simulink model "STATCOM_Model"  (R2017a)
settings: Solver=FixedStepDiscrete  StartTime=0.0  StopTime=3  RelTol=1e-4  EnableMultiTasking=on
PreLoadFcn:
  | power_converters_init;
values from neighbouring files (symbols this model uses):
  Clink_3L = Pnom_dc_3L*H_3L*2 /Vnom_dc_3L^2    (= 2.77008310249e-05)    [STATCOM_init.m]
  Fnom = 50    [STATCOM_init.m]
  LimitL_Ireg_3L = -1.5    [STATCOM_init.m]
  LimitU_Ireg_3L = 1.5    [STATCOM_init.m]
  Lxfo_3L = 0.10    (= 0.1)    [STATCOM_init.m]
  Pnom_3L = Pnom_dc_3L    (= 50000000)    [STATCOM_init.m]
  Pnom_dc_3L = 50e6    (= 50000000)    [STATCOM_init.m]
  Rxfo_3L = 0.10/30    (= 0.00333333333333)    [STATCOM_init.m]
  Ts_Control = 50e-6    (= 5e-05)    [STATCOM_init.m]
  Ts_Power = Ts_PWM    (= 5e-06)    [STATCOM_init.m]
  Ts_PWM = 5e-6    (= 5e-06)    [STATCOM_init.m]
  Vnom_dc_3L = 380e3    (= 380000)    [STATCOM_init.m]
  Vnom_grid = 230e3    (= 230000)    [STATCOM_init.m]
  Vnom_prim_3L = Vnom_grid    (= 230000)    [STATCOM_init.m]
  Vnom_sec_3L = 0.5*Vnom_dc_3L/sqrt(2)*sqrt(3)*m_nom_3L    [STATCOM_init.m]
undefined symbols (not defined in the file or in its folder): D1, Delta, DiscIntNeverNeededParam
undefined symbols (not defined in the file): Ki_Ireg_3L, Ki_VDCreg_3L, Kp_Ireg_3L, Kp_VDCreg_3L, LimitL_VDCreg_3L, LimitU_VDCreg_3L
libraries: powerlib x23, powerlib_meascontrol x11, powerlib_extras x1
(part 2 of 2)

== system STATCOM_Model/Control System  ==
  Statcom Control : Subsystem

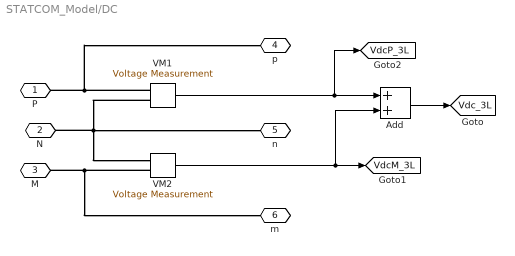
== system STATCOM_Model/DC ==
  Add : Sum
  VM1 : powerlib/Measurements/Voltage Measurement  PhasorSimulation=off  OutputType=Complex  PSBequivalent=0
  VM2 : powerlib/Measurements/Voltage Measurement  PhasorSimulation=off  OutputType=Complex  PSBequivalent=0
  P : PMIOPort  Port=1  Side=Left
  N : PMIOPort  Port=2  Side=Left
  M : PMIOPort  Port=3  Side=Left
  p : PMIOPort  Port=4  Side=Right
  n : PMIOPort  Port=5  Side=Right
  m : PMIOPort  Port=6  Side=Right
  tag scope: VdcM_3L=global, VdcP_3L=global, Vdc_3L=global
  wires:
  VM1/1 -> [VdcP_3L], Add/1
  VM2/1 -> Add/2, [VdcM_3L]
  Add/1 -> [Vdc_3L]
  connections:
  VM1/LConn1 -- p/RConn1 -- P/RConn1
  VM2/LConn2 -- m/RConn1 -- M/RConn1
  VM1/LConn2 -- n/RConn1 -- VM2/LConn1 -- N/RConn1

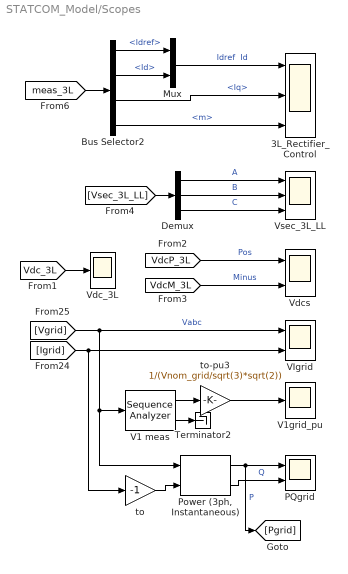
== system STATCOM_Model/Scopes ==
  3L_Rectifier_Control : Scope  NumInputPorts=3
  Bus Selector2 : BusSelector  OutputSignals=Idref,Id,Iq,m
  Demux : Demux  Outputs=3
  Mux : Mux  Inputs=2
  PQgrid : Scope  NumInputPorts=2
  "Power (3ph, Instantaneous)" : powerlib_meascontrol/Measurements/Power (3ph, Instantaneous)
      settings: SourceProductName=Simscape Power Systems
  Terminator2 : Terminator
  V1 meas : powerlib_meascontrol/Measurements/Sequence Analyzer  Freq=Fnom  n=1  seq=Positive  InInit=[1, 0]  Ts=Ts_Power
      settings: SourceProductName=Simscape Power Systems  SourceProductBaseCode=PS
  V1grid_pu : Scope
  VIgrid : Scope  NumInputPorts=2
  Vdc_3L : Scope
  Vdcs : Scope  NumInputPorts=2
  Vsec_3L_LL : Scope  NumInputPorts=3
  to : Gain  Gain=-1
  to-pu3 : Gain  Gain=1/(Vnom_grid/sqrt(3)*sqrt(2))
  wires:
  [meas_3L] -> Bus Selector2/1
  "Power (3ph, Instantaneous)"/1 -> [Pgrid], PQgrid/1  "P"
  V1 meas/2 -> Terminator2/1
  V1 meas/1 -> to-pu3/1
  to-pu3/1 -> V1grid_pu/1
  Mux/1 -> 3L_Rectifier_Control/1  "Idref  Id"
  Bus Selector2/1 -> Mux/1  "<Idref>"
  Bus Selector2/2 -> Mux/2  "<Id>"
  Bus Selector2/4 -> 3L_Rectifier_Control/3  "<m>"
  Bus Selector2/3 -> 3L_Rectifier_Control/2  "<Iq>"
  [Vdc_3L] -> Vdc_3L/1
  [VdcP_3L] -> Vdcs/1  "Pos"
  [VdcM_3L] -> Vdcs/2  "Minus"
  [Vsec_3L_LL] -> Demux/1
  Demux/1 -> Vsec_3L_LL/1  "A"
  Demux/2 -> Vsec_3L_LL/2  "B"
  Demux/3 -> Vsec_3L_LL/3  "C"
  "Power (3ph, Instantaneous)"/2 -> PQgrid/2  "Q"
  to/1 -> "Power (3ph, Instantaneous)"/2
  [Igrid] -> VIgrid/2, to/1
  [Vgrid] -> VIgrid/1, "Power (3ph, Instantaneous)"/1, V1 meas/1  "Vabc"

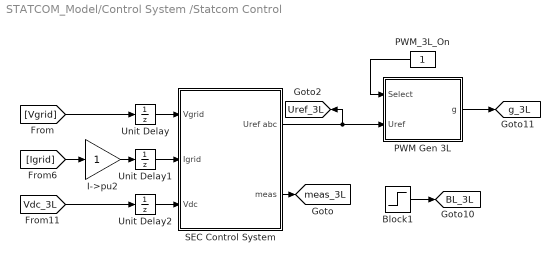
== system STATCOM_Model/Control System /Statcom Control ==
  Block1 : Step  Time=999  SampleTime=Ts_Power
  I->pu2 : Gain  SaturateOnIntegerOverflow=on  OutDataTypeStr=Inherit: Same as input  ParamDataTypeStr=Inherit: Same as input
  PWM Gen 3L : Subsystem
  PWM_3L_On : Constant
      settings: AttributesFormatString=%<Tag>
  SEC Control System : Subsystem
  Unit Delay : UnitDelay  SampleTime=Ts_Power
  Unit Delay1 : UnitDelay  SampleTime=Ts_Power
  Unit Delay2 : UnitDelay  SampleTime=Ts_Power
  tag scope: BL_3L=global, Uref_3L=global, g_3L=global, meas_3L=global
  wires:
  SEC Control System/2(meas) -> [meas_3L]
  Block1/1 -> [BL_3L]
  [Vgrid] -> Unit Delay/1
  SEC Control System/1(Uref abc) -> [Uref_3L], PWM Gen 3L/2(Uref)
  [Vdc_3L] -> Unit Delay2/1
  Unit Delay1/1 -> SEC Control System/2(Igrid)
  Unit Delay2/1 -> SEC Control System/3(Vdc)
  Unit Delay/1 -> SEC Control System/1(Vgrid)
  PWM Gen 3L/1(g) -> [g_3L]
  PWM_3L_On/1 -> PWM Gen 3L/1(Select)
  I->pu2/1 -> Unit Delay1/1
  [Igrid] -> I->pu2/1

== system STATCOM_Model/Control System /Statcom Control/PWM Gen 3L ==
  Select : Inport
  Uref : Inport  Port=2
  PWMgen - Averaging : Subsystem
  Pavg_3L : Subsystem
  Switch : Switch  Threshold=1.5
  g : Outport
  wires:
  Select/1 -> PWMgen - Averaging/Enable, Switch/2
  PWMgen - Averaging/1(g1_avg) -> Pavg_3L/1(g1)
  Switch/1 -> g/1
  PWMgen - Averaging/2(g4_avg) -> Pavg_3L/2(g4)
  PWMgen - Averaging/3(P) -> Switch/3
  Uref/1 -> PWMgen - Averaging/1(Uref)
  Pavg_3L/1(g) -> Switch/1

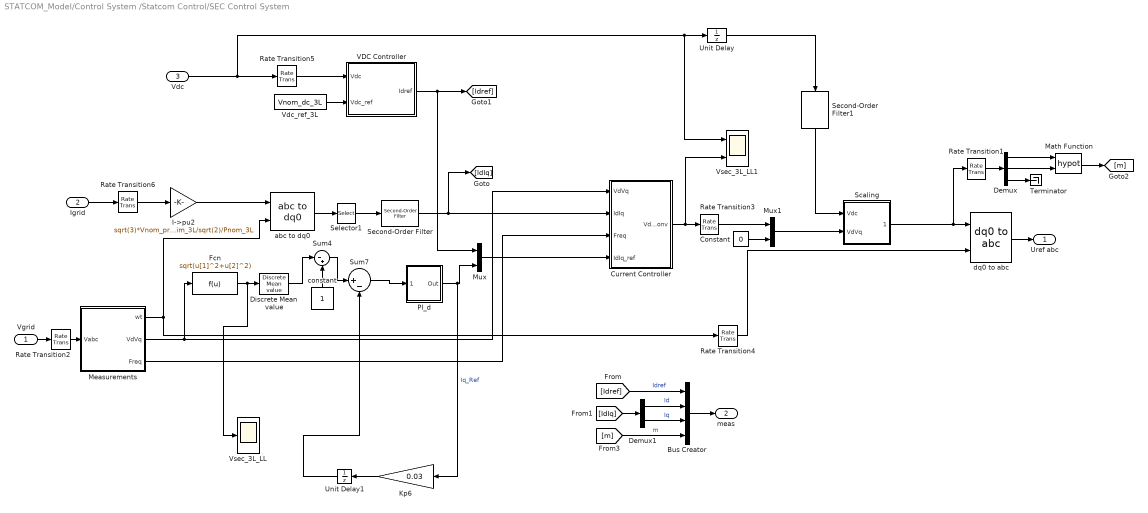
== system STATCOM_Model/Control System /Statcom Control/SEC Control System ==
  Vgrid : Inport  PortDimensions=3
  Igrid : Inport  Port=2  PortDimensions=3
  Vdc : Inport  Port=3
  Bus Creator : BusCreator  Inputs=4
  Constant : Constant  Value=0
  Current Controller : Subsystem
  Demux : Demux  Outputs=3
  Demux1 : Demux  Outputs=2
  Discrete Mean value : powerlib_extras/Discrete Measurements/Discrete  Mean value  Freq=60  Vinit=1  Ts=Ts_Control
  Fcn : Fcn  Expr=sqrt(u[1]^2+u[2]^2)  SampleTime=Ts_Control
  I->pu2 : Gain  Gain=sqrt(3)*Vnom_prim_3L/sqrt(2)/Pnom_3L  SaturateOnIntegerOverflow=on  OutDataTypeStr=Inherit: Same as input  ParamDataTypeStr=Inherit: Same as input
  Kp6 : Gain  Gain=0.03  SaturateOnIntegerOverflow=on  OutDataTypeStr=Inherit: Same as input  ParamDataTypeStr=Inherit: Same as input
  Math Function : Math  Operator=hypot  SaturateOnIntegerOverflow=on
  Measurements : Subsystem
  Mux : Mux  Inputs=2
  Mux1 : Mux  Inputs=[2 1]
  PI_d : Subsystem  DialogController=POWERSYS.PowerSysDialog  mask(Discrete PI Controller){Kp=0.5, Ki=50, Par_Limits=[1  -1], Init=0, Ts=Ts_Control}
      mask prompts: Kp "Proportional gain (Kp):"; Ki "Integral gain (Ki):"; Par_Limits "Output limits: [ Upper   Lower ]"; Init "Output initial value:"; Ts "Sample time:"
      mask help: This block implements a discrete PI controller.
      mask init:
      | UpperLimit=Par_Limits(1);
      | LowerLimit=Par_Limits(2);
      mask Display: disp('PI');
  Rate Transition{1..2,5..6} (4 alike) : RateTransition  OutPortSampleTime=Ts_Control
  Rate Transition3 : RateTransition  OutPortSampleTime=Ts_PWM
  Rate Transition4 : RateTransition  OutPortSampleTime=Ts_PWM
  Scaling : Subsystem
  Second-Order Filter : powerlib_meascontrol/Filters/Second-Order Filter  FilterType=Lowpass  Fo=Freq_Filter  Zeta=1  Ts=Ts_Control  Initialize=off  Vac_Init="[0,  0,  60]"  Vdc_Init=0  PlotResponse=off  FreqRange=[0, 500, 1]
      settings: SourceProductName=Simscape Power Systems  SourceProductBaseCode=PS
  Second-Order Filter1 : powerlib_meascontrol/Filters/Second-Order Filter  FilterType=Lowpass  Fo=Freq_Filter  Zeta=1  Ts=Ts_PWM  Initialize=off  Vac_Init="[0,  0,  60]"  Vdc_Init=0  PlotResponse=off  FreqRange=[0, 500, 1]
      settings: SourceProductName=Simscape Power Systems  SourceProductBaseCode=PS
  Selector1 : Selector  InputPortWidth=3  IndexOptions=Index vector (dialog)  Indices=[1 2]  OutputSizes=1
  Sum4 : Sum  Inputs=|-+
  Sum7 : Sum  Inputs=|+-  SaturateOnIntegerOverflow=on  InputSameDT=on  OutDataTypeStr=Inherit: Same as first input
  Terminator : Terminator
  Unit Delay : UnitDelay  SampleTime=Ts_PWM
  Unit Delay1 : UnitDelay  SampleTime=Ts_Control
  VDC Controller : Subsystem
  Vdc_ref_3L : Constant  Value=Vnom_dc_3L
  Vsec_3L_LL : Scope
  Vsec_3L_LL1 : Scope  NumInputPorts=2
  abc to dq0 : powerlib_meascontrol/Transformations/abc to dq0  Alignment=90 degrees behind phase A axis
  constant : Constant  SampleTime=Ts_Control
  dq0 to abc : powerlib_meascontrol/Transformations/dq0 to abc  Alignment=90 degrees behind phase A axis
  Uref abc : Outport
  meas : Outport  Port=2
  wires:
  Selector1/1 -> Second-Order Filter/1
  I->pu2/1 -> abc to dq0/1
  Igrid/1 -> Rate Transition6/1
  abc to dq0/1 -> Selector1/1
  VDC Controller/1(Idref) -> [Idref], Mux/1
  Scaling/1(VdVq*) -> dq0 to abc/1, Rate Transition1/1
  Mux1/1 -> Scaling/2(VdVq)
  Mux/1 -> Current Controller/4(IdIq_ref)
  Demux/3 -> Terminator/1
  Demux/2 -> Math Function/2
  Demux/1 -> Math Function/1
  Constant/1 -> Mux1/2
  Rate Transition3/1 -> Mux1/1
  Rate Transition4/1 -> dq0 to abc/2
  Current Controller/1(VdVq_conv) -> Vsec_3L_LL1/2, Rate Transition3/1
  dq0 to abc/1 -> Uref abc/1
  Vgrid/1 -> Rate Transition2/1
  Rate Transition2/1 -> Measurements/1(Vabc)
  Rate Transition6/1 -> I->pu2/1
  Measurements/1(wt) -> Rate Transition4/1, abc to dq0/2
  Measurements/2(VdVq) -> Current Controller/1(VdVq), Fcn/1
  Measurements/3(Freq) -> Current Controller/3(Freq)
  Vdc_ref_3L/1 -> VDC Controller/2(Vdc_ref)
  [Idref] -> Bus Creator/1  "Idref"
  Demux1/1 -> Bus Creator/2  "Id"
  Demux1/2 -> Bus Creator/3  "Iq"
  [m] -> Bus Creator/4  "m"
  [IdIq] -> Demux1/1
  Bus Creator/1 -> meas/1
  Math Function/1 -> [m]
  Rate Transition5/1 -> VDC Controller/1(Vdc)
  Rate Transition1/1 -> Demux/1
  Vdc/1 -> Vsec_3L_LL1/1, Unit Delay/1, Rate Transition5/1
  Unit Delay/1 -> Second-Order Filter1/1
  Second-Order Filter/1 -> [IdIq], Current Controller/2(IdIq)
  Second-Order Filter1/1 -> Scaling/1(Vdc)
  Discrete Mean value/1 -> Sum4/1
  constant/1 -> Sum4/2
  Unit Delay1/1 -> Sum7/2
  Kp6/1 -> Unit Delay1/1
  PI_d/1(Out) -> Kp6/1, Mux/2  "Iq_Ref"
  Sum4/1 -> Sum7/1
  Sum7/1 -> PI_d/1(Error)
  Fcn/1 -> Vsec_3L_LL/1, Discrete Mean value/1

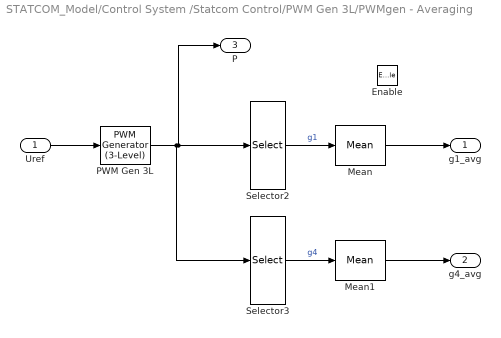
== system STATCOM_Model/Control System /Statcom Control/PWM Gen 3L/PWMgen - Averaging ==
  Uref : Inport
  Enable : EnablePort
  Mean : powerlib_meascontrol/Measurements/Mean  Freq=1/Ts_Power  Vinit=0  Ts=Ts_PWM
  Mean1 : powerlib_meascontrol/Measurements/Mean  Freq=1/Ts_Power  Vinit=0  Ts=Ts_PWM
  PWM Gen 3L : powerlib_meascontrol/Pulse & Signal Generators/PWM Generator (3-Level)  ModulatorType=Three-phase bridge (12 pulses)  ModulatorMode=Unsynchronized  nF=27  Fc=Fc_3L  ModulatingSignals=off  m=0.8  Freq=60  Phase=0  Ts=Ts_PWM
      settings: SourceProductName=Simscape Power Systems  SourceProductBaseCode=PS
  Selector2 : Selector  InputPortWidth=12  IndexOptions=Index vector (dialog)  Indices="[1  5  9]"  OutputSizes=1
  Selector3 : Selector  InputPortWidth=12  IndexOptions=Index vector (dialog)  Indices="[1  5  9]+3"  OutputSizes=1
  g1_avg : Outport
  g4_avg : Outport  Port=2
  P : Outport  Port=3
  wires:
  Uref/1 -> PWM Gen 3L/1
  PWM Gen 3L/1 -> P/1, Selector2/1, Selector3/1
  Selector3/1 -> Mean1/1  "g4"
  Selector2/1 -> Mean/1  "g1"
  Mean/1 -> g1_avg/1
  Mean1/1 -> g4_avg/1

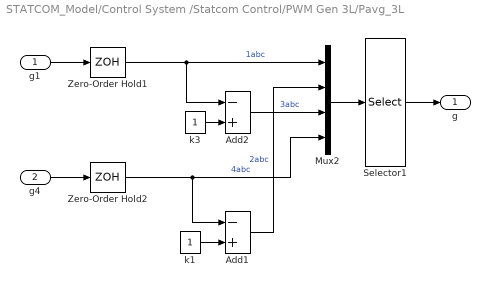
== system STATCOM_Model/Control System /Statcom Control/PWM Gen 3L/Pavg_3L ==
  g1 : Inport  SampleTime=Ts_PWM
  g4 : Inport  Port=2  SampleTime=Ts_PWM
  Add1 : Sum  Inputs=-+
  Add2 : Sum  Inputs=-+
  Mux2 : Mux  Inputs=[ 3 3 3 3 ]
  Selector1 : Selector  InputPortWidth=12  IndexOptions=Index vector (dialog)  Indices=[1 4 7 10 2 5 8 11 3 6 9 12]  OutputSizes=1
  Zero-Order Hold1 : ZeroOrderHold  SampleTime=Ts_Power
  Zero-Order Hold2 : ZeroOrderHold  SampleTime=Ts_Power
  k1 : Constant
  k3 : Constant
  g : Outport  SampleTime=Ts_Power
  wires:
  Selector1/1 -> g/1
  Mux2/1 -> Selector1/1
  Add1/1 -> Mux2/2  "2abc"
  Add2/1 -> Mux2/3  "3abc"
  Zero-Order Hold2/1 -> Mux2/4, Add1/1  "4abc"
  k1/1 -> Add1/2
  Zero-Order Hold1/1 -> Mux2/1, Add2/1  "1abc"
  k3/1 -> Add2/2
  g1/1 -> Zero-Order Hold1/1
  g4/1 -> Zero-Order Hold2/1

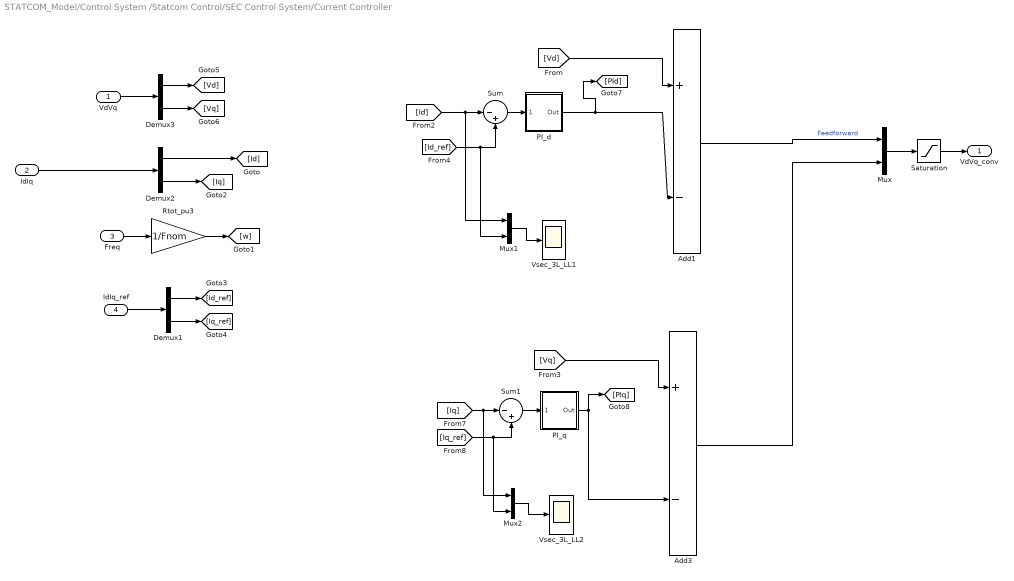
== system STATCOM_Model/Control System /Statcom Control/SEC Control System/Current Controller ==
  VdVq : Inport  PortDimensions=2
  IdIq : Inport  Port=2  PortDimensions=2
  Freq : Inport  Port=3  PortDimensions=1
  IdIq_ref : Inport  Port=4  PortDimensions=2
  Add1 : Sum  Inputs=+-
  Add3 : Sum  Inputs=+-
  Demux1 : Demux  Outputs=2
  Demux2 : Demux  Outputs=2
  Demux3 : Demux  Outputs=2
  Mux : Mux  Inputs=2
  Mux1 : Mux  Inputs=2
  Mux2 : Mux  Inputs=2
  PI_d : Subsystem  DialogController=POWERSYS.PowerSysDialog  mask(Discrete PI Controller){Kp=Kp_Ireg_3L, Ki=Ki_Ireg_3L, Par_Limits=[ LimitU_Ireg_3L LimitL_Ireg_3L ], Init=0, Ts=Ts_Control}
      mask prompts: Kp "Proportional gain (Kp):"; Ki "Integral gain (Ki):"; Par_Limits "Output limits: [ Upper   Lower ]"; Init "Output initial value:"; Ts "Sample time:"
      mask help: This block implements a discrete PI controller.
      mask init:
      | UpperLimit=Par_Limits(1);
      | LowerLimit=Par_Limits(2);
      mask Display: disp('PI');
  PI_q : Subsystem  DialogController=POWERSYS.PowerSysDialog  mask(Discrete PI Controller){Kp=Kp_Ireg_3L, Ki=Ki_Ireg_3L, Par_Limits=[ LimitU_Ireg_3L LimitL_Ireg_3L ], Init=0, Ts=Ts_Control}
      mask prompts: Kp "Proportional gain (Kp):"; Ki "Integral gain (Ki):"; Par_Limits "Output limits: [ Upper   Lower ]"; Init "Output initial value:"; Ts "Sample time:"
      mask help: This block implements a discrete PI controller.
      mask init:
      | UpperLimit=Par_Limits(1);
      | LowerLimit=Par_Limits(2);
      mask Display: disp('PI');
  Rtot_pu3 : Gain  Gain=1/Fnom  SaturateOnIntegerOverflow=on  OutDataTypeStr=Inherit: Same as input  ParamDataTypeStr=Inherit: Same as input
  Saturation : Saturate  UpperLimit=LimitU_Ireg_3L  LowerLimit=LimitL_Ireg_3L
  Sum : Sum  Inputs=|-+
  Sum1 : Sum  Inputs=|-+
  Vsec_3L_LL1 : Scope
  Vsec_3L_LL2 : Scope
  VdVq_conv : Outport
  wires:
  Add1/1 -> Mux/1  "Feedforward"
  PI_d/1(Out) -> [PId], Add1/2
  PI_q/1(Out) -> [PIq], Add3/2
  [Vd] -> Add1/1
  [Vq] -> Add3/1
  Demux2/1 -> [Id]
  IdIq/1 -> Demux2/1
  Saturation/1 -> VdVq_conv/1
  [Id] -> Mux1/1, Sum/1
  [Iq] -> Mux2/1, Sum1/1
  Demux2/2 -> [Iq]
  Add3/1 -> Mux/2
  [Iq_ref] -> Mux2/2, Sum1/2
  Sum1/1 -> PI_q/1(Error)
  [Id_ref] -> Mux1/2, Sum/2
  Sum/1 -> PI_d/1(Error)
  Mux/1 -> Saturation/1
  VdVq/1 -> Demux3/1
  Demux3/2 -> [Vq]
  Demux3/1 -> [Vd]
  IdIq_ref/1 -> Demux1/1
  Demux1/2 -> [Iq_ref]
  Demux1/1 -> [Id_ref]
  Rtot_pu3/1 -> [w]
  Freq/1 -> Rtot_pu3/1
  Mux1/1 -> Vsec_3L_LL1/1
  Mux2/1 -> Vsec_3L_LL2/1

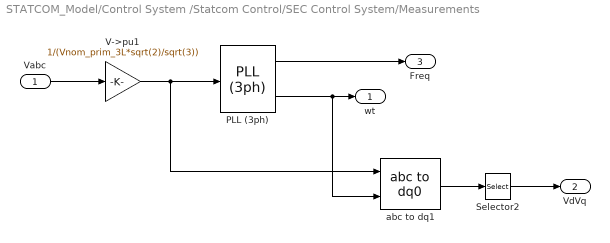
== system STATCOM_Model/Control System /Statcom Control/SEC Control System/Measurements ==
  Vabc : Inport  PortDimensions=3
  PLL (3ph) : powerlib_meascontrol/PLL/PLL (3ph)  Fmin=45  Par_Init=[0, Fnom]  ParK=[180, 3200, 0]/2  TcD=1e-4  MaxRateChangeFreq=12  FilterCutOffFreq=25  Ts=Ts_Control  AGC=on
  Selector2 : Selector  InputPortWidth=3  IndexOptions=Index vector (dialog)  Indices=[1 2]  OutputSizes=1
  V->pu1 : Gain  Gain=1/(Vnom_prim_3L*sqrt(2)/sqrt(3))  SaturateOnIntegerOverflow=on  OutDataTypeStr=Inherit: Same as input  ParamDataTypeStr=Inherit: Same as input
  abc to dq1 : powerlib_meascontrol/Transformations/abc to dq0  Alignment=90 degrees behind phase A axis
  wt : Outport
  VdVq : Outport  Port=2
  Freq : Outport  Port=3
  wires:
  Selector2/1 -> VdVq/1
  abc to dq1/1 -> Selector2/1
  PLL (3ph)/1 -> Freq/1
  V->pu1/1 -> PLL (3ph)/1, abc to dq1/1
  Vabc/1 -> V->pu1/1
  PLL (3ph)/2 -> wt/1, abc to dq1/2

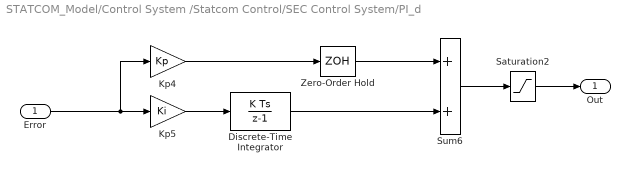
== system STATCOM_Model/Control System /Statcom Control/SEC Control System/PI_d ==
  Error : Inport  SampleTime=Ts
  Discrete-Time Integrator : DiscreteIntegrator  InitialCondition=Init  SampleTime=Ts  LimitOutput=on  UpperSaturationLimit=UpperLimit  LowerSaturationLimit=LowerLimit  ICPrevOutput=DiscIntNeverNeededParam  ICPrevScaledInput=DiscIntNeverNeededParam
  Kp4 : Gain  Gain=Kp  SampleTime=Ts  SaturateOnIntegerOverflow=on  OutDataTypeStr=Inherit: Same as input  ParamDataTypeStr=Inherit: Same as input
  Kp5 : Gain  Gain=Ki  SampleTime=Ts  SaturateOnIntegerOverflow=on  OutDataTypeStr=Inherit: Same as input  ParamDataTypeStr=Inherit: Same as input
  Saturation2 : Saturate  UpperLimit=UpperLimit  LowerLimit=LowerLimit  SampleTime=Ts
  Sum6 : Sum  SampleTime=Ts  SaturateOnIntegerOverflow=on  InputSameDT=on  OutDataTypeStr=Inherit: Same as first input
  Zero-Order Hold : ZeroOrderHold  SampleTime=Ts
  Out : Outport  SampleTime=Ts  InitialOutput=0
  wires:
  Saturation2/1 -> Out/1
  Error/1 -> Kp4/1, Kp5/1
  Sum6/1 -> Saturation2/1
  Kp5/1 -> Discrete-Time Integrator/1
  Kp4/1 -> Zero-Order Hold/1
  Discrete-Time Integrator/1 -> Sum6/2
  Zero-Order Hold/1 -> Sum6/1

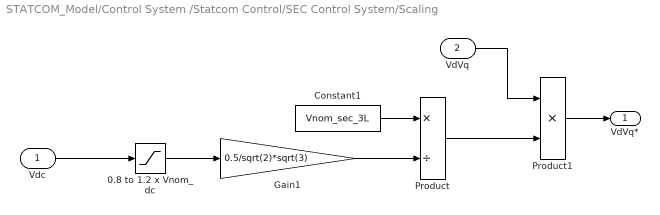
== system STATCOM_Model/Control System /Statcom Control/SEC Control System/Scaling ==
  Vdc : Inport
  VdVq : Inport  Port=2
  0.8 to 1.2 x Vnom_dc : Saturate  UpperLimit=1.5*Vnom_dc_3L  LowerLimit=0.5*Vnom_dc_3L
  Constant1 : Constant  Value=Vnom_sec_3L
  Gain1 : Gain  Gain=0.5/sqrt(2)*sqrt(3)
  Product : Product  Inputs=*/
  Product1 : Product  Inputs=**
  VdVq* : Outport
  wires:
  Product1/1 -> VdVq*/1
  VdVq/1 -> Product1/1
  Vdc/1 -> 0.8 to 1.2 x Vnom_dc/1
  Product/1 -> Product1/2
  0.8 to 1.2 x Vnom_dc/1 -> Gain1/1
  Gain1/1 -> Product/2
  Constant1/1 -> Product/1

== system STATCOM_Model/Control System /Statcom Control/SEC Control System/VDC Controller ==
  Vdc : Inport  PortDimensions=1
  Vdc_ref : Inport  Port=2  PortDimensions=1
  Gain : Gain  Gain=1/(Vnom_dc_3L)
  PI_d : Subsystem  DialogController=POWERSYS.PowerSysDialog  mask(Discrete PI Controller){Kp=Kp_VDCreg_3L, Ki=Ki_VDCreg_3L, Par_Limits=[ LimitU_VDCreg_3L LimitL_VDCreg_3L ], Init=0, Ts=Ts_Control}
      mask prompts: Kp "Proportional gain (Kp):"; Ki "Integral gain (Ki):"; Par_Limits "Output limits: [ Upper   Lower ]"; Init "Output initial value:"; Ts "Sample time:"
      mask help: This block implements a discrete PI controller.
      mask init:
      | UpperLimit=Par_Limits(1);
      | LowerLimit=Par_Limits(2);
      mask Display: disp('PI');
  Sum : Sum  Inputs=|+-
  Idref : Outport
  wires:
  PI_d/1(Out) -> Idref/1
  Gain/1 -> PI_d/1(Error)
  Vdc/1 -> Sum/2
  Vdc_ref/1 -> Sum/1
  Sum/1 -> Gain/1

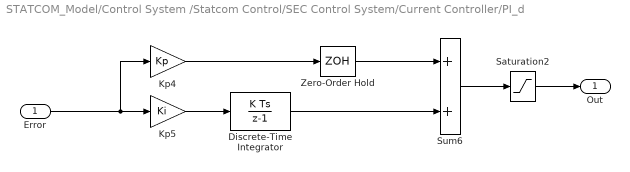
== system STATCOM_Model/Control System /Statcom Control/SEC Control System/Current Controller/PI_d ==
  Error : Inport  SampleTime=Ts
  Discrete-Time Integrator : DiscreteIntegrator  InitialCondition=Init  SampleTime=Ts  LimitOutput=on  UpperSaturationLimit=UpperLimit  LowerSaturationLimit=LowerLimit  ICPrevOutput=DiscIntNeverNeededParam  ICPrevScaledInput=DiscIntNeverNeededParam
  Kp4 : Gain  Gain=Kp  SampleTime=Ts  SaturateOnIntegerOverflow=on  OutDataTypeStr=Inherit: Same as input  ParamDataTypeStr=Inherit: Same as input
  Kp5 : Gain  Gain=Ki  SampleTime=Ts  SaturateOnIntegerOverflow=on  OutDataTypeStr=Inherit: Same as input  ParamDataTypeStr=Inherit: Same as input
  Saturation2 : Saturate  UpperLimit=UpperLimit  LowerLimit=LowerLimit  SampleTime=Ts
  Sum6 : Sum  SampleTime=Ts  SaturateOnIntegerOverflow=on  InputSameDT=on  OutDataTypeStr=Inherit: Same as first input
  Zero-Order Hold : ZeroOrderHold  SampleTime=Ts
  Out : Outport  SampleTime=Ts  InitialOutput=0
  wires:
  Saturation2/1 -> Out/1
  Error/1 -> Kp4/1, Kp5/1
  Sum6/1 -> Saturation2/1
  Kp5/1 -> Discrete-Time Integrator/1
  Kp4/1 -> Zero-Order Hold/1
  Discrete-Time Integrator/1 -> Sum6/2
  Zero-Order Hold/1 -> Sum6/1

== system STATCOM_Model/Control System /Statcom Control/SEC Control System/Current Controller/PI_q ==
  Error : Inport  SampleTime=Ts
  Discrete-Time Integrator : DiscreteIntegrator  InitialCondition=Init  SampleTime=Ts  LimitOutput=on  UpperSaturationLimit=UpperLimit  LowerSaturationLimit=LowerLimit  ICPrevOutput=DiscIntNeverNeededParam  ICPrevScaledInput=DiscIntNeverNeededParam
  Kp4 : Gain  Gain=Kp  SampleTime=Ts  SaturateOnIntegerOverflow=on  OutDataTypeStr=Inherit: Same as input  ParamDataTypeStr=Inherit: Same as input
  Kp5 : Gain  Gain=Ki  SampleTime=Ts  SaturateOnIntegerOverflow=on  OutDataTypeStr=Inherit: Same as input  ParamDataTypeStr=Inherit: Same as input
  Saturation2 : Saturate  UpperLimit=UpperLimit  LowerLimit=LowerLimit  SampleTime=Ts
  Sum6 : Sum  SampleTime=Ts  SaturateOnIntegerOverflow=on  InputSameDT=on  OutDataTypeStr=Inherit: Same as first input
  Zero-Order Hold : ZeroOrderHold  SampleTime=Ts
  Out : Outport  SampleTime=Ts  InitialOutput=0
  wires:
  Zero-Order Hold/1 -> Sum6/1
  Discrete-Time Integrator/1 -> Sum6/2
  Kp4/1 -> Zero-Order Hold/1
  Kp5/1 -> Discrete-Time Integrator/1
  Sum6/1 -> Saturation2/1
  Error/1 -> Kp5/1, Kp4/1
  Saturation2/1 -> Out/1

== system STATCOM_Model/Control System /Statcom Control/SEC Control System/VDC Controller/PI_d ==
  Error : Inport  SampleTime=Ts
  Discrete-Time Integrator : DiscreteIntegrator  InitialCondition=Init  SampleTime=Ts  LimitOutput=on  UpperSaturationLimit=UpperLimit  LowerSaturationLimit=LowerLimit  ICPrevOutput=DiscIntNeverNeededParam  ICPrevScaledInput=DiscIntNeverNeededParam
  Kp4 : Gain  Gain=Kp  SampleTime=Ts  SaturateOnIntegerOverflow=on  OutDataTypeStr=Inherit: Same as input  ParamDataTypeStr=Inherit: Same as input
  Kp5 : Gain  Gain=Ki  SampleTime=Ts  SaturateOnIntegerOverflow=on  OutDataTypeStr=Inherit: Same as input  ParamDataTypeStr=Inherit: Same as input
  Saturation2 : Saturate  UpperLimit=UpperLimit  LowerLimit=LowerLimit  SampleTime=Ts
  Sum6 : Sum  SampleTime=Ts  SaturateOnIntegerOverflow=on  InputSameDT=on  OutDataTypeStr=Inherit: Same as first input
  Zero-Order Hold : ZeroOrderHold  SampleTime=Ts
  Out : Outport  SampleTime=Ts  InitialOutput=0
  wires:
  Saturation2/1 -> Out/1
  Error/1 -> Kp4/1, Kp5/1
  Sum6/1 -> Saturation2/1
  Kp5/1 -> Discrete-Time Integrator/1
  Kp4/1 -> Zero-Order Hold/1
  Discrete-Time Integrator/1 -> Sum6/2
  Zero-Order Hold/1 -> Sum6/1
